simulink model "HARV_6DoF_turn_mdl"  (Simulink 9.3)
settings: Solver=ode45  StartTime=0.0  StopTime=100  FixedStep=0.01  MaxStep=0.01  MinStep=0.000001  RelTol=1e-3
model workspace (MAT data in the model file):
  op_trim1 : opcond.OperatingReport (value not decoded)
  op_trim3 : opcond.OperatingReport (value not decoded)
  op_trim5 : opcond.OperatingReport (value not decoded)
values from neighbouring files (symbols this model uses):
  b = 37.42*0.305    (= 11.4131)    [HARV_model.m]
  cbar = 11.52*0.305    (= 3.5136)    [HARV_model.m]
  GM = [c3 0 c4 0 c2 0 0 c1 0 ... (first row only)    [HARV_model.m]
  m = 1128.09*14.5939    (= 16463.232651)    [HARV_model.m]
  S = 400*(0.305^2)    (= 37.21)    [HARV_model.m]
undefined symbols (not defined in the file or in its folder): ad, ae, airlib, B747, DT, eqm, fms, gr, hlp
libraries: simulink x1
(part 1 of 2)
settings Model: Creator=kumabhi  LastModifiedBy=kumabhi
settings SolverCC: InitialStep=0.001  SolverJacobianMethodControl=SparsePerturbation
settings DataIOCC: ExternalInput=getinputstruct(op3)  InitialState=getstatestruct(op3)  LoadExternalInput=on  LoadInitialState=on  SignalLoggingSaveFormat=Dataset  SaveState=on  ReturnWorkspaceOutputs=on
settings OptimizationCC: LifeSpan=auto
settings DebuggingCC: UnderspecifiedInitializationDetection=Simplified  MergeDetectMultiDrivingBlocksExec=error  FcnCallInpInsideContextMsg=error  SFUnexpectedBacktrackingDiag=error  SFNoUnconditionalDefaultTransitionDiag=error  SFExecutionAtInitializationDiag=warning  ArithmeticOperatorsInVariantConditions=error
settings HardwareCC: ProdBitPerPointer=64  ProdBitPerSizeT=64  ProdBitPerPtrDiffT=64  ProdLargestAtomicFloat=Float  ProdIntDivRoundTo=Zero  ProdEndianess=LittleEndian  ProdWordSize=64  ProdHWDeviceType=Intel->x86-64 (Windows64)
settings ModelReferenceCC: PropagateSignalLabelsOutOfModel=on
settings SFSimCC: SimUseLocalCustomCode=on
settings RTWCC: RTWUseLocalCustomCode=on
settings CodeAppCC: StateflowObjectComments=off
settings GRTTargetCC: TargetLangStandard=C99 (ISO)  CombineOutputUpdateFcns=on  GRTInterface=off
settings ConfigComp: CovMetricSettings=dwe  CovHtmlReporting=off  CovSaveCumulativeToWorkspaceVar=off  CovSaveSingleToWorkspaceVar=off  CovExternalEMLEnable=on

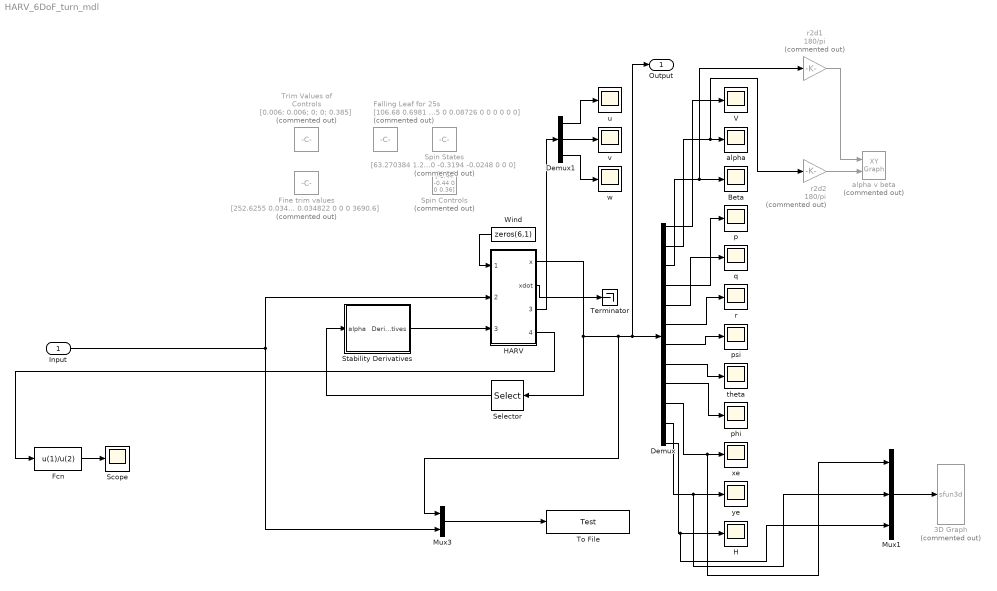
== system HARV_6DoF_turn_mdl ==
  Input : Inport
  3D Graph : S-Function  Commented=on  LoadFcn=if exist('sfun3d','file'), sfun3d([],[],[],'LoadBlock'); end  FunctionName=sfun3d  Parameters=ax,T,np,cp,gd,ls,mk,mx,hd,tb  SFunctionDeploymentMode=off  EnableBusSupport=off  mask(3D Graph){np=1, ax=[-300 3000 -3000 3000 -3000 3000], mx=1e7, T=0.1, cp=[3 2 1], gd=on, hd=off, tb=off, ls=-, mk=none}
      mask prompts: np "Number of moving points (lines)"; ax "Range: [xmin xmax  ymin ymax zmin zmax]"; mx "Max number of points in each line"; T "Sampling Time"; cp "Camera position (use [0 0 1] for 2D XY view)"; gd "Grid (on|off)"; hd "HeadMarkers (on|off)"; tb "Toolbar (on|off)"; ls "LineStyle"; mk "LineMarker"
      mask help:
      | This block plots the position of several points in the XYZ space. The input contains the coordinates of all the points (x1,y1,z1,x2,y2,z2,...).
      | The number of moving points (lines), the XYZ ranges, sampling time, camera position, and grid (among other things) can be set as mask parameters.
      settings: CopyFcn=if exist('sfun3d','file'), sfun3d([],[],[],'CopyBlock'); end  DeleteFcn=if exist('sfun3d','file'), sfun3d([],[],[],'DeleteBlock'); end  NameChangeFcn=if exist('sfun3d','file'), sfun3d([],[],[],'NameChange'); end
      mask Help:
      | This block plots the position of several points in the XYZ space. The input contains the coordinates of all the points (x1,y1,z1,x2,y2,z2,...).
      | The number of moving points (lines), the XYZ ranges, sampling time, camera position, and grid (among other things) can be set as mask parameters.
      mask TypeOptions ls: - | -- | : | -. | none
      mask TypeOptions mk: none | . | + | o | * | x | square | diamond | v | ^ | > | < | pentagram | hexagram
      mask Display: plot([.05 .95 .95 .05 .05],[.45 .45 .95 .95 .45], 0.5+cos(0:0.1:2*pi)*0.3,0.7+sin(0:0.1:2*pi)*0.2)
  Beta : Scope
  Demux : Demux  Outputs=12
  Demux1 : Demux  Outputs=3
  Falling Leaf for 25s : Constant  Commented=on  Value=[106.68 0.6981 0.349 0.1745 0 0.08726 0 0 0 0 0 0]
  Fcn : Fcn  Expr=u(1)/u(2)
  "Fine trim values " : Constant  Commented=on  Value=[252.6255 0.03482432 0 0 0 0 0 0.034822 0 0 0 3690.6]
  H : Scope
  HARV : Subsystem  AncestorBlock=airlib/DT-B747
  Mux1 : Mux  Inputs=3
  Mux3 : Mux  Inputs=2
  Scope : Scope
  Selector : Selector  InputPortWidth=12  IndexOptions=Index vector (dialog)  Indices=[2]  OutputSizes=1
  "Spin Controls " : Constant  Commented=on  Value=[-0.44 -0.44 0 0 0.36]
  "Spin States " : Constant  Commented=on  Value=[63.270384 1.2375 0.0382 -0.6163 0.1784 -1.4645 0 -0.3194 -0.0248 0 0 0]
  Stability Derivatives : Subsystem
  Terminator : Terminator
  To File : ToFile  Filename=Test  SaveFormat=Timeseries
  "Trim Values of Controls " : Constant  Commented=on  Value=[0.006; 0.006; 0; 0; 0.385]
  V : Scope
  Wind : Constant  Value=zeros(6,1)
  alpha : Scope
  alpha v beta : simulink/Sinks/XY Graph  Commented=on  xmin=-75  xmax=75  ymin=-30  ymax=80  st=-1
  p : Scope
  phi : Scope
  psi : Scope
  q : Scope
  r : Scope
  r2d1 : Gain  Commented=on  Gain=180/pi
  r2d2 : Gain  Commented=on  Gain=180/pi
  theta : Scope
  u : Scope
  v : Scope
  w : Scope
  xe : Scope
  ye : Scope
  Output : Outport
  wires:
  HARV/1(x) -> Mux3/1, Output/1, Demux/1, Selector/1
  Wind/1 -> HARV/1(Wind)
  Demux/1 -> V/1
  Demux/2 -> r2d2/1, alpha/1
  Demux/3 -> r2d1/1, Beta/1
  Demux/4 -> p/1
  Demux/5 -> q/1
  Demux/6 -> r/1
  Demux/7 -> psi/1
  Demux/8 -> theta/1
  Demux/11 -> Mux1/2, ye/1
  Demux/12 -> Mux1/3, H/1
  Demux/9 -> phi/1
  Demux/10 -> Mux1/1, xe/1
  HARV/3("[u v w]") -> Demux1/1
  Demux1/1 -> u/1
  Demux1/2 -> v/1
  Demux1/3 -> w/1
  HARV/2(xdot) -> Terminator/1
  Selector/1 -> Stability Derivatives/1(alpha)
  Stability Derivatives/1(Derivatives) -> HARV/3(Stability Derivatives)
  Mux1/1 -> 3D Graph/1
  r2d2/1 -> alpha v beta/2
  r2d1/1 -> alpha v beta/1
  Mux3/1 -> To File/1
  HARV/4(CAero) -> Fcn/1
  Input/1 -> HARV/2(Control), Mux3/2
  Fcn/1 -> Scope/1

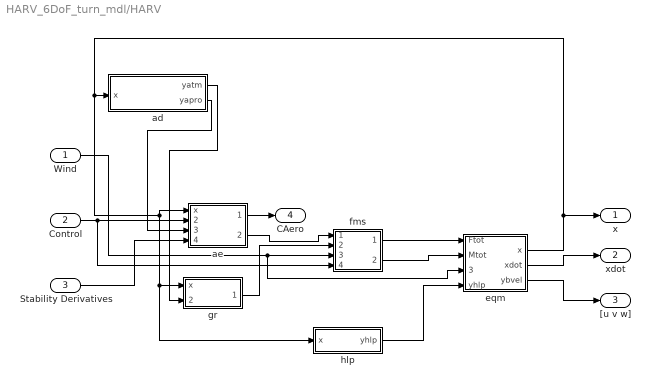
== system HARV_6DoF_turn_mdl/HARV ==
  Wind : Inport
  Control : Inport  Port=2
  Stability Derivatives : Inport  Port=3
  ad : Subsystem  AncestorBlock=airlib/DT-B747/ad
      mask Display: disp('ATMOSPHERE')
  ae : Subsystem  AncestorBlock=airlib/DT-B747/ae
      mask Display: disp('Faero')
  eqm : Subsystem  AncestorBlock=airlib/DT-B747/eqm
      mask Display: disp('ODE')
  fms : Subsystem  AncestorBlock=airlib/DT-B747/fms  mask(FMsort){}
      mask help: Forces and Moments sorting block
      mask Display: disp('FMsort')
  gr : Subsystem  AncestorBlock=airlib/DT-B747/gr  mask(Gravity){m=m}
      mask prompts: m "Mass of the aircraft [kg]:"
      mask help: Gravity forces.
      mask Display: disp('Gravity')
  hlp : Subsystem  AncestorBlock=airlib/DT-B747/hlp  mask(Hlpfcn){}
      mask help: Help sines and cosines
      mask Display: disp('hlpfcn')
  x : Outport
  xdot : Outport  Port=2
  "[u v w]" : Outport  Port=3
  CAero : Outport  Port=4
  wires:
  ad/2(yapro) -> ae/3(yaprop)
  Control/1 -> fms/4(Control), ae/2(Control)
  Stability Derivatives/1 -> ae/4(Stability Derivatives)
  ad/1(yatm) -> gr/2(yatm)
  ae/2(FMaero) -> fms/1(FMaero)
  Wind/1 -> eqm/3(uwind), fms/3(Fwind)
  gr/1(Fgrav) -> fms/2(Fgrav)
  ae/1(Caero) -> CAero/1
  fms/1(Ftot) -> eqm/1(Ftot)
  fms/2(Mtot) -> eqm/2(Mtot)
  hlp/1(yhlp) -> eqm/4(yhlp)
  eqm/1(x) -> hlp/1(x), gr/1(x), ae/1(x), ad/1(x), x/1
  eqm/2(xdot) -> xdot/1
  eqm/3(ybvel) -> "[u v w]"/1

== system HARV_6DoF_turn_mdl/Stability Derivatives ==
  alpha : Inport
  Lateral : Subsystem
  Longitudinal : Subsystem
  Mux : Mux  Inputs=2
  Derivatives : Outport
  wires:
  alpha/1 -> Longitudinal/1(alpha), Lateral/1(alpha)
  Lateral/1("CY, Cl, Cn") -> Mux/1
  Longitudinal/1("CL, CD, CM") -> Mux/2
  Mux/1 -> Derivatives/1

== system HARV_6DoF_turn_mdl/HARV/ad ==
  x : Inport
  ad1 : Subsystem  mask(Airdata1){}
      mask help: Basic airdata variables
      mask Display: disp('Airdata1')
  atm : Subsystem  mask(Atmosph){}
      mask help: Atmosphere variables
      mask Display: disp('Atmosph')
  yatm : Outport
  yapro : Outport  Port=2
  wires:
  ad1/1(yap) -> yapro/1
  atm/1(yatm) -> ad1/2(yatm), yatm/1
  x/1 -> ad1/1(x), atm/1(x)

== system HARV_6DoF_turn_mdl/HARV/ae ==
  x : Inport
  Control : Inport  Port=2
  yaprop : Inport  Port=3
  Stability Derivatives : Inport  Port=4
  ae : Subsystem  Commented=on  AncestorBlock=airlib/DT-B747/ae
  ae1 : Subsystem  AncestorBlock=airlib/DT-B747/ae
  ae2 : Subsystem  AncestorBlock=airlib/DT-B747/ae
  fmdims : Subsystem
      mask Display: disp('Forces & Moments')
  hlp : Subsystem  AncestorBlock=airlib/DT-B747/hlp  mask(Hlpfcn){}
      mask help: Help sines and cosines
      mask Display: disp('hlpfcn')
  Caero : Outport
  FMaero : Outport  Port=2
  wires:
  fmdims/1(Forces and moments) -> FMaero/1
  yaprop/1 -> ae2/2(ya), fmdims/1(yad1)
  Control/1 -> ae2/3(Controls)
  Stability Derivatives/1 -> ae2/1(Stability Derivatives)
  x/1 -> ae2/4(x), hlp/1(x)
  ae2/1(Output) -> ae1/1(Caero), Caero/1
  hlp/1(yhlp) -> ae1/2(helpfcn)
  ae1/1(CForce) -> fmdims/2(Force / moment derivatives)

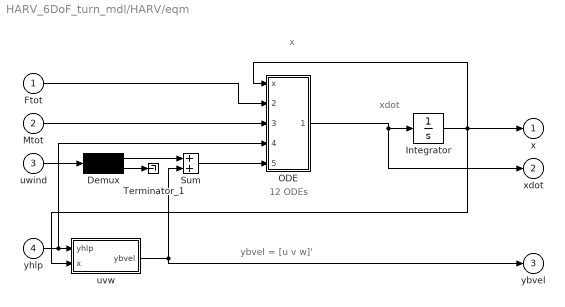
== system HARV_6DoF_turn_mdl/HARV/eqm ==
  note: 12 ODEs
  note: ybvel = [u v w]'
  note: x
  note: xdot
  Ftot : Inport
  Mtot : Inport  Port=2
  uwind : Inport  Port=3
  yhlp : Inport  Port=4
  Demux : Demux  Outputs=[3 3]
  Integrator : Integrator  InitialCondition=[54.7 0.5 0 -0.109 0.678 0.0538 0 0.9 0.9 0 0 0]
  ODE : Subsystem
  Sum : Sum  SaturateOnIntegerOverflow=on  InputSameDT=on  OutDataTypeStr=Inherit: Same as first input
  Terminator_1 : Terminator
  uvw : Subsystem  mask(uvw){}
      mask help:
      | Calculation of body-axes velocities
      | u, v, and w
      mask Display: disp('Body-axes\nvelocities')
  x : Outport
  xdot : Outport  Port=2
  ybvel : Outport  Port=3
  wires:
  ODE/1(xdot) -> Integrator/1, xdot/1
  Integrator/1 -> uvw/2(x), ODE/1(x), x/1
  Mtot/1 -> ODE/3(Mtot)
  Ftot/1 -> ODE/2(Ftot)
  Demux/1 -> Sum/1
  uwind/1 -> Demux/1
  uvw/1(ybvel) -> Sum/2, ybvel/1
  Sum/1 -> ODE/5(ybvel*)
  yhlp/1 -> ODE/4(yhlp), uvw/1(yhlp)
  Demux/2 -> Terminator_1/1

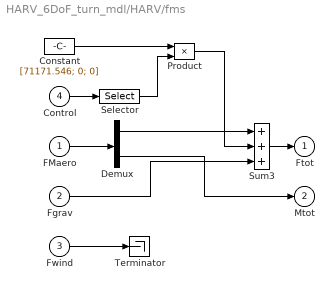
== system HARV_6DoF_turn_mdl/HARV/fms ==
  FMaero : Inport
  Fgrav : Inport  Port=2
  Fwind : Inport  Port=3
  Control : Inport  Port=4
  Constant : Constant  Value=[71171.546; 0; 0]
  Demux : Demux  Outputs=[3 3]
  Product : Product
  Selector : Selector  InputPortWidth=5  IndexOptions=Index vector (dialog)  Indices=[5]  OutputSizes=1
  Sum3 : Sum  Inputs=+++  SaturateOnIntegerOverflow=on  InputSameDT=on  OutDataTypeStr=Inherit: Same as first input
  Terminator : Terminator
  Ftot : Outport
  Mtot : Outport  Port=2
  wires:
  Demux/1 -> Sum3/1
  Demux/2 -> Mtot/1
  Sum3/1 -> Ftot/1
  Fgrav/1 -> Sum3/3
  FMaero/1 -> Demux/1
  Fwind/1 -> Terminator/1
  Control/1 -> Selector/1
  Selector/1 -> Product/2
  Constant/1 -> Product/1
  Product/1 -> Sum3/2

== system HARV_6DoF_turn_mdl/HARV/gr ==
  x : Inport
  yatm : Inport  Port=2
  Mux : Mux  Inputs=3
  Mux1 : Mux  Inputs=[12 5]
  Xgr : Fcn  Expr=-m*u[17]*sin(u[8])
  Ygr : Fcn  Expr=m*u[17]*cos(u[8])*sin(u[9])
  Zgr : Fcn  Expr=m*u[17]*cos(u[8])*cos(u[9])
  Fgrav : Outport
  wires:
  yatm/1 -> Mux1/2
  x/1 -> Mux1/1
  Zgr/1 -> Mux/3
  Mux1/1 -> Zgr/1, Xgr/1, Ygr/1
  Mux/1 -> Fgrav/1
  Ygr/1 -> Mux/2
  Xgr/1 -> Mux/1

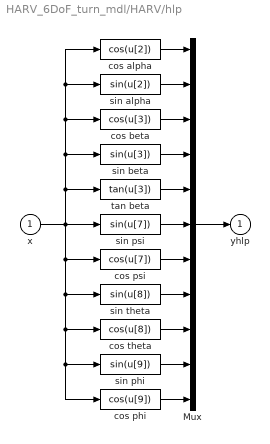
== system HARV_6DoF_turn_mdl/HARV/hlp ==
  x : Inport
  Mux : Mux  Inputs=11
  cos alpha : Fcn  Expr=cos(u[2])
  cos beta : Fcn  Expr=cos(u[3])
  cos phi : Fcn  Expr=cos(u[9])
  cos psi : Fcn  Expr=cos(u[7])
  cos theta : Fcn  Expr=cos(u[8])
  sin alpha : Fcn  Expr=sin(u[2])
  sin beta : Fcn  Expr=sin(u[3])
  sin phi : Fcn  Expr=sin(u[9])
  sin psi : Fcn  Expr=sin(u[7])
  sin theta : Fcn  Expr=sin(u[8])
  tan beta : Fcn  Expr=tan(u[3])
  yhlp : Outport
  wires:
  cos phi/1 -> Mux/11
  Mux/1 -> yhlp/1
  sin phi/1 -> Mux/10
  cos theta/1 -> Mux/9
  sin theta/1 -> Mux/8
  cos psi/1 -> Mux/7
  sin psi/1 -> Mux/6
  tan beta/1 -> Mux/5
  sin beta/1 -> Mux/4
  cos beta/1 -> Mux/3
  sin alpha/1 -> Mux/2
  cos alpha/1 -> Mux/1
  x/1 -> cos psi/1, cos phi/1, sin phi/1, cos theta/1, sin theta/1, tan beta/1, cos alpha/1, sin alpha/1, cos beta/1, sin beta/1, sin psi/1

== system HARV_6DoF_turn_mdl/Stability Derivatives/Lateral ==
  alpha : Inport
  CY : Subsystem
  Cl : Subsystem
  Cn : Subsystem
  Mux : Mux  Inputs=3
  "CY, Cl, Cn" : Outport
  wires:
  alpha/1 -> Cn/1(alpha), Cl/1(alpha), CY/1(alpha)
  Mux/1 -> "CY, Cl, Cn"/1
  CY/1(CY) -> Mux/1
  Cl/1(Cl) -> Mux/2
  Cn/1(Cn) -> Mux/3

== system HARV_6DoF_turn_mdl/Stability Derivatives/Longitudinal ==
  alpha : Inport
  CD : Subsystem
  CL : Subsystem
  CM : Subsystem
  Mux : Mux  Inputs=3
  "CL, CD, CM" : Outport
  wires:
  alpha/1 -> CD/1(Input), CL/1(alpha), CM/1(Input)
  CD/1(Output) -> Mux/1
  CL/1(CL_derivatives) -> Mux/2
  CM/1(Output) -> Mux/3
  Mux/1 -> "CL, CD, CM"/1

== system HARV_6DoF_turn_mdl/HARV/ad/ad1 ==
  x : Inport
  yatm : Inport  Port=2
  M : Fcn  Expr=u[2]/u[1]
  Mux : Mux  Inputs=[1 12]
  Mux1 : Mux  Inputs=[12 5]
  Mux2 : Mux  Inputs=3
  a : Fcn  Expr=sqrt(401.8743*u[3])
  qdyn : Fcn  Expr=0.5*u[13]*u[1]^2
  yap : Outport
  wires:
  yatm/1 -> Mux1/2, a/1
  x/1 -> Mux1/1, Mux/2
  Mux/1 -> M/1
  Mux1/1 -> qdyn/1
  M/1 -> Mux2/2
  a/1 -> Mux2/1, Mux/1
  qdyn/1 -> Mux2/3
  Mux2/1 -> yap/1

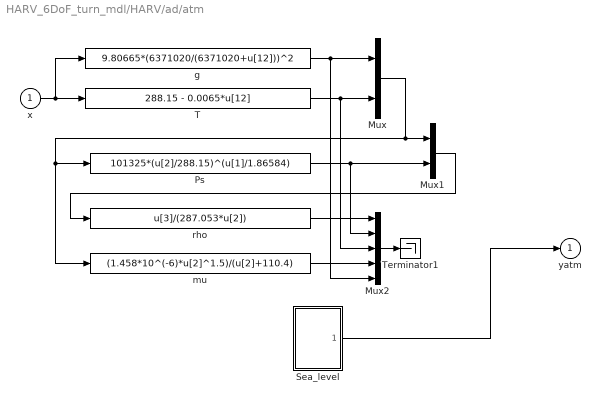
== system HARV_6DoF_turn_mdl/HARV/ad/atm ==
  x : Inport
  Mux : Mux  Inputs=2
  Mux1 : Mux  Inputs=[2 1]
  Mux2 : Mux  Inputs=5
  Ps : Fcn  Expr=101325*(u[2]/288.15)^(u[1]/1.86584)
  Sea_level : Subsystem
  T : Fcn  Expr=288.15 - 0.0065*u[12]
  Terminator1 : Terminator
  g : Fcn  Expr=9.80665*(6371020/(6371020+u[12]))^2
  mu : Fcn  Expr=(1.458*10^(-6)*u[2]^1.5)/(u[2]+110.4)
  rho : Fcn  Expr=u[3]/(287.053*u[2])
  yatm : Outport
  wires:
  mu/1 -> Mux2/4
  Mux1/1 -> rho/1
  rho/1 -> Mux2/1
  g/1 -> Mux2/5, Mux/1
  T/1 -> Mux2/3, Mux/2
  Ps/1 -> Mux2/2, Mux1/2
  Mux/1 -> Ps/1, mu/1, Mux1/1
  x/1 -> g/1, T/1
  Mux2/1 -> Terminator1/1
  Sea_level/1(Sea Level) -> yatm/1

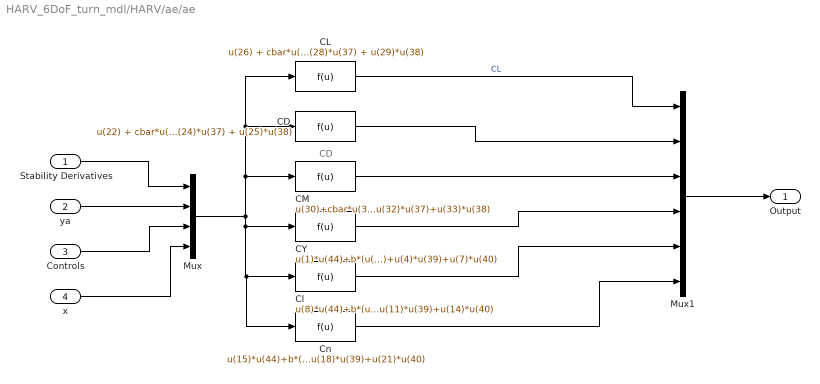
== system HARV_6DoF_turn_mdl/HARV/ae/ae ==
  note: CD
  Stability Derivatives : Inport
  ya : Inport  Port=2
  Controls : Inport  Port=3
  x : Inport  Port=4
  CD : Fcn  Expr=u(22) + cbar*u(23)*u(46)/(2*u(42))+ u(24)*u(37) + u(25)*u(38)
  CL : Fcn  Expr=u(26) + cbar*u(27)*u(46)/(2*u(42))+ u(28)*u(37) + u(29)*u(38)
  CM : Fcn  Expr=u(30)+cbar*u(31)*u(46)/(2*u(42))+u(32)*u(37)+u(33)*u(38)
  CY : Fcn  Expr=u(1)*u(44)+b*(u(2)*u(45)+u(3)*u(47))/(2*u(42))+u(4)*u(39)+u(7)*u(40)
  Cl : Fcn  Expr=u(8)*u(44)+b*(u(9)*u(45)+u(10)*u(47))/(2*u(42))+u(11)*u(39)+u(14)*u(40)
  Cn : Fcn  Expr=u(15)*u(44)+b*(u(16)*u(45)+u(17)*u(47))/(2*u(42))+u(18)*u(39)+u(21)*u(40)
  Mux : Mux
  Mux1 : Mux  Inputs=6
  Output : Outport
  wires:
  Stability Derivatives/1 -> Mux/1
  ya/1 -> Mux/2
  Mux/1 -> CM/1, CD/1, CL/1, Cn/1, Cl/1, CY/1
  Controls/1 -> Mux/3
  x/1 -> Mux/4
  CL/1 -> Mux1/1  "CL"
  CD/1 -> Mux1/2
  CM/1 -> Mux1/3
  CY/1 -> Mux1/4
  Cl/1 -> Mux1/5
  Cn/1 -> Mux1/6
  Mux1/1 -> Output/1

== system HARV_6DoF_turn_mdl/HARV/ae/ae1 ==
  Caero : Inport
  helpfcn : Inport  Port=2
  CX : Fcn  Expr=-u(2)*u(7)+u(1)*u(8)
  CZ : Fcn  Expr=-u(2)*u(8)-u(1)*u(7)
  Demux : Demux
  Mux : Mux  Inputs=2
  Mux1 : Mux  Inputs=6
  Selector : Selector  InputPortWidth=17  IndexOptions=Index vector (dialog)  Indices=[3:6]  OutputSizes=1
  CForce : Outport
  wires:
  Caero/1 -> Mux/1
  helpfcn/1 -> Mux/2
  Mux/1 -> Selector/1, CZ/1, CX/1
  CX/1 -> Mux1/1
  Mux1/1 -> CForce/1
  Selector/1 -> Demux/1
  CZ/1 -> Mux1/3
  Demux/2 -> Mux1/2
  Demux/3 -> Mux1/4
  Demux/1 -> Mux1/5
  Demux/4 -> Mux1/6

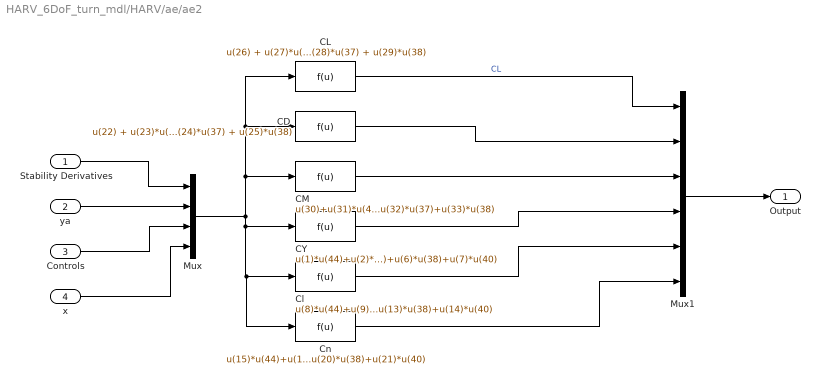
== system HARV_6DoF_turn_mdl/HARV/ae/ae2 ==
  Stability Derivatives : Inport
  ya : Inport  Port=2
  Controls : Inport  Port=3
  x : Inport  Port=4
  CD : Fcn  Expr=u(22) + u(23)*u(46)+ u(24)*u(37) + u(25)*u(38)
  CL : Fcn  Expr=u(26) + u(27)*u(46)+ u(28)*u(37) + u(29)*u(38)
  CM : Fcn  Expr=u(30)+u(31)*u(46)+u(32)*u(37)+u(33)*u(38)
  CY : Fcn  Expr=u(1)*u(44)+u(2)*u(45)+u(3)*u(47)+u(4)*u(39)+u(5)*u(37)+u(6)*u(38)+u(7)*u(40)
  Cl : Fcn  Expr=u(8)*u(44)+u(9)*u(45)+u(10)*u(47)+u(11)*u(39)+u(12)*u(37)+u(13)*u(38)+u(14)*u(40)
  Cn : Fcn  Expr=u(15)*u(44)+u(16)*u(45)+u(17)*u(47)+u(18)*u(39)+u(19)*u(37)+u(20)*u(38)+u(21)*u(40)
  Mux : Mux
  Mux1 : Mux  Inputs=6
  Output : Outport
  wires:
  Stability Derivatives/1 -> Mux/1
  ya/1 -> Mux/2
  Mux/1 -> CM/1, CD/1, CL/1, Cn/1, Cl/1, CY/1
  Controls/1 -> Mux/3
  x/1 -> Mux/4
  CL/1 -> Mux1/1  "CL"
  CD/1 -> Mux1/2
  CM/1 -> Mux1/3
  CY/1 -> Mux1/4
  Cl/1 -> Mux1/5
  Cn/1 -> Mux1/6
  Mux1/1 -> Output/1

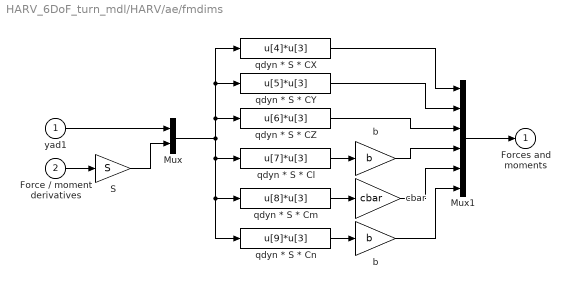
== system HARV_6DoF_turn_mdl/HARV/ae/fmdims ==
  yad1 : Inport
  Force / moment derivatives : Inport  Port=2
  Mux : Mux  Inputs=[3 6]
  Mux1 : Mux  Inputs=6
  S : Gain  Gain=S  SaturateOnIntegerOverflow=on  OutDataTypeStr=Inherit: Same as input  ParamDataTypeStr=Inherit: Same as input
  b : Gain  Gain=b  SaturateOnIntegerOverflow=on  OutDataTypeStr=Inherit: Same as input  ParamDataTypeStr=Inherit: Same as input
  "b " : Gain  Gain=b  SaturateOnIntegerOverflow=on  OutDataTypeStr=Inherit: Same as input  ParamDataTypeStr=Inherit: Same as input
  cbar : Gain  Gain=cbar  SaturateOnIntegerOverflow=on  OutDataTypeStr=Inherit: Same as input  ParamDataTypeStr=Inherit: Same as input
  qdyn * S * CX : Fcn  Expr=u[4]*u[3]
  qdyn * S * CY : Fcn  Expr=u[5]*u[3]
  qdyn * S * CZ : Fcn  Expr=u[6]*u[3]
  qdyn * S * Cl : Fcn  Expr=u[7]*u[3]
  qdyn * S * Cm : Fcn  Expr=u[8]*u[3]
  qdyn * S * Cn : Fcn  Expr=u[9]*u[3]
  Forces and moments : Outport
  wires:
  b/1 -> Mux1/4
  qdyn * S * CZ/1 -> Mux1/3
  S/1 -> Mux/2
  qdyn * S * CY/1 -> Mux1/2
  qdyn * S * CX/1 -> Mux1/1
  yad1/1 -> Mux/1
  qdyn * S * Cn/1 -> "b "/1
  qdyn * S * Cm/1 -> cbar/1
  qdyn * S * Cl/1 -> b/1
  Mux/1 -> qdyn * S * Cn/1, qdyn * S * Cm/1, qdyn * S * Cl/1, qdyn * S * CY/1, qdyn * S * CX/1, qdyn * S * CZ/1
  Force / moment derivatives/1 -> S/1
  cbar/1 -> Mux1/5
  "b "/1 -> Mux1/6
  Mux1/1 -> Forces and moments/1

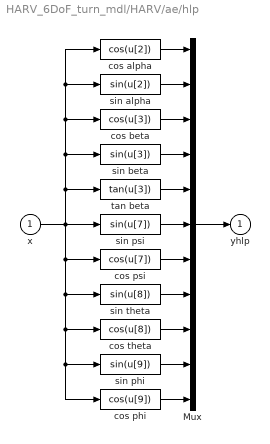
== system HARV_6DoF_turn_mdl/HARV/ae/hlp ==
  x : Inport
  Mux : Mux  Inputs=11
  cos alpha : Fcn  Expr=cos(u[2])
  cos beta : Fcn  Expr=cos(u[3])
  cos phi : Fcn  Expr=cos(u[9])
  cos psi : Fcn  Expr=cos(u[7])
  cos theta : Fcn  Expr=cos(u[8])
  sin alpha : Fcn  Expr=sin(u[2])
  sin beta : Fcn  Expr=sin(u[3])
  sin phi : Fcn  Expr=sin(u[9])
  sin psi : Fcn  Expr=sin(u[7])
  sin theta : Fcn  Expr=sin(u[8])
  tan beta : Fcn  Expr=tan(u[3])
  yhlp : Outport
  wires:
  cos phi/1 -> Mux/11
  Mux/1 -> yhlp/1
  sin phi/1 -> Mux/10
  cos theta/1 -> Mux/9
  sin theta/1 -> Mux/8
  cos psi/1 -> Mux/7
  sin psi/1 -> Mux/6
  tan beta/1 -> Mux/5
  sin beta/1 -> Mux/4
  cos beta/1 -> Mux/3
  sin alpha/1 -> Mux/2
  cos alpha/1 -> Mux/1
  x/1 -> cos psi/1, cos phi/1, sin phi/1, cos theta/1, sin theta/1, tan beta/1, cos alpha/1, sin alpha/1, cos beta/1, sin beta/1, sin psi/1

== system HARV_6DoF_turn_mdl/HARV/eqm/ODE ==
  x : Inport
  Ftot : Inport  Port=2
  Mtot : Inport  Port=3
  yhlp : Inport  Port=4
  ybvel* : Inport  Port=5
  Eulerdot : Subsystem  mask(Eulerdot){}
      mask help:
      | Calculation of d(psi)/dt, d(theta)/dt,
      | and d(phi/dt)
      mask Display: disp('psi dot\ntheta dot\nphi dot')
  Mux : Mux  Inputs=[12 3 3 11]
  Mux1 : Mux  Inputs=[3 3 3 3]
  Vabdot : Subsystem  mask(Vabdot){}
      mask help: Calculation of dV/dt, dalpha/dt, dbeta/dt.
      mask Display: disp('V dot\nalpha dot\nbeta dot')
  pqrdot : Subsystem  mask(pqrdot){}
      mask help: Calculation of dp/dt, dq/dt, and dr/dt
      mask Display: disp('p dot\nq dot\nr dot')
  xyHdot : Subsystem  mask(xyHdot){}
      mask help: Calculation of d(xe)/dt, d(ye)/dt, and dH/dt
      mask Display: disp('xe dot\nye dot\nH dot')
  xdot : Outport
  wires:
  Mux1/1 -> xdot/1
  Vabdot/1(yVab) -> Mux1/1
  pqrdot/1(ypqr) -> Mux1/2
  Eulerdot/1(yeul) -> Mux1/3
  xyHdot/1(yxyH) -> Mux1/4
  yhlp/1 -> Mux/4
  ybvel*/1 -> xyHdot/1(ybvel*)
  Mux/1 -> xyHdot/2(uxYH), Eulerdot/1(ueul), Vabdot/1(uVab), pqrdot/1(upqr)
  Ftot/1 -> Mux/2
  Mtot/1 -> Mux/3
  x/1 -> Mux/1

== system HARV_6DoF_turn_mdl/HARV/eqm/uvw ==
  yhlp : Inport
  x : Inport  Port=2
  Mux : Mux  Inputs=3
  Mux1 : Mux  Inputs=[12 11]
  u : Fcn  Expr=u[1]*u[13]*u[15]
  v : Fcn  Expr=u[1]*u[16]
  w : Fcn  Expr=u[1]*u[14]*u[15]
  ybvel : Outport
  wires:
  Mux/1 -> ybvel/1
  w/1 -> Mux/3
  v/1 -> Mux/2
  u/1 -> Mux/1
  x/1 -> Mux1/1
  yhlp/1 -> Mux1/2
  Mux1/1 -> v/1, w/1, u/1

== system HARV_6DoF_turn_mdl/Stability Derivatives/Lateral/CY ==
  alpha : Inport
  CY_b : Lookup_n-D  NumberOfTableDimensions=1  BreakpointsForDimension1=[-0.2444,-0.1746,-0.1048,-0.0349,0.0349,0.1048,0.1746,0.2444,0.3143,0.3841,0.4540,0.5238,0.5937,0.6635,0.7333,0.8032,0.8730,0.9429,1.0127,1.0825,1.1524,1.2222,1.2921,1.3619,1.4317,1.5016,1.5714]  Table=[-0.9848,-0.9848,-1.0161,-1.0473,-1.0549,-1.0547,-1.0754,-1.0145,-0.8881,-0.8074,-0.7265,-0.7373,-0.7168,-0.7766,-0.8036,-0.7625,-0.6844,0.7484,-0.7853,-0.7877,-0.7642,-0.7393,-0.7622,-0.7922,-0.7893,-0.7544,-0.7294]  InternalRulePriority=Speed  RndMeth=Simplest  InputSameDT=on
  CY_da : Lookup_n-D  NumberOfTableDimensions=1  BreakpointsForDimension1=[-0.2444,-0.1746,-0.1048,-0.0349,0.0349,0.1048,0.1746,0.2444,0.3143,0.3841,0.4540,0.5238,0.5937,0.6635,0.7333,0.8032,0.8730,0.9429,1.0127,1.0825,1.1524,1.2222,1.2921,1.3619,1.4317,1.5016,1.5714]  Table=|  InternalRulePriority=Speed  RndMeth=Simplest  InputSameDT=on
      | [
      |    -0.0331,
      |    -0.0331,
      |    -0.0331,
      |    -0.0313,
      |    -0.0264,
      |    -0.0233,
      |    -0.0238,
      |    -0.0212,
      |    -0.0112,
      |     0.0026,
      |     0.0151,
      |     0.0271,
      |     0.0366,
      |     0.0406,
      |     0.0372,
      |     0.0114,
      |    -0.0058,
      |    -0.0085,
      |    -0.0100,
      |    -0.0112,
      |    -0.0125,
      |    -0.0138,
      |    -0.0159,
      |    -0.0175,
      |    -0.0188,
      |    -0.0199,
      |    -0.0210]
  CY_da1 : Lookup_n-D  Commented=on  NumberOfTableDimensions=1  BreakpointsForDimension1=[-0.2444,-0.1746,-0.1048,-0.0349,0.0349,0.1048,0.1746,0.2444,0.3143,0.3841,0.4540,0.5238,0.5937,0.6635,0.7333,0.8032,0.8730,0.9429,1.0127,1.0825,1.1524,1.2222,1.2921,1.3619,1.4317,1.5016,1.5714]  Table=[0,0,0,0,0,0,0,0,0,0,0,0,0,0,0,0,0,0,0,0,0,0,0,0,0,0,0]  InternalRulePriority=Speed  RndMeth=Simplest  InputSameDT=on
  CY_del : Lookup_n-D  NumberOfTableDimensions=1  BreakpointsForDimension1=[-0.2444,-0.1746,-0.1048,-0.0349,0.0349,0.1048,0.1746,0.2444,0.3143,0.3841,0.4540,0.5238,0.5937,0.6635,0.7333,0.8032,0.8730,0.9429,1.0127,1.0825,1.1524,1.2222,1.2921,1.3619,1.4317,1.5016,1.5714]  Table=|  InternalRulePriority=Speed  RndMeth=Simplest  InputSameDT=on
      | [   -0.0698,
      |    -0.0698,
      |    -0.0698,
      |    -0.0679,
      |    -0.0622,
      |    -0.0555,
      |    -0.0494,
      |    -0.0403,
      |    -0.0286,
      |    -0.0165,
      |    -0.0029,
      |     0.0118,
      |     0.0245,
      |     0.0339,
      |     0.0416,
      |     0.0491,
      |     0.0576,
      |     0.0648,
      |     0.0703,
      |     0.0747,
      |     0.0743,
      |     0.0616,
      |     0.0289,
      |    -0.0026,
      |    -0.0326,
      |    -0.0573,
      |    -0.0693]
  CY_der : Lookup_n-D  NumberOfTableDimensions=1  BreakpointsForDimension1=[-0.2444,-0.1746,-0.1048,-0.0349,0.0349,0.1048,0.1746,0.2444,0.3143,0.3841,0.4540,0.5238,0.5937,0.6635,0.7333,0.8032,0.8730,0.9429,1.0127,1.0825,1.1524,1.2222,1.2921,1.3619,1.4317,1.5016,1.5714]  Table=|  InternalRulePriority=Speed  RndMeth=Simplest  InputSameDT=on
      | [    0.0698,
      |     0.0698,
      |     0.0698,
      |     0.0679,
      |     0.0622,
      |     0.0555,
      |     0.0494,
      |     0.0403,
      |     0.0286,
      |     0.0165,
      |     0.0029,
      |    -0.0118,
      |    -0.0245,
      |    -0.0339,
      |    -0.0416,
      |    -0.0491,
      |    -0.0576,
      |    -0.0648,
      |    -0.0703,
      |    -0.0747,
      |    -0.0743,
      |    -0.0616,
      |    -0.0289,
      |     0.0026,
      |     0.0326,
      |     0.0573,
      |     0.0693]
  CY_dr : Lookup_n-D  NumberOfTableDimensions=1  BreakpointsForDimension1=[-0.2444,-0.1746,-0.1048,-0.0349,0.0349,0.1048,0.1746,0.2444,0.3143,0.3841,0.4540,0.5238,0.5937,0.6635,0.7333,0.8032,0.8730,0.9429,1.0127,1.0825,1.1524,1.2222,1.2921,1.3619,1.4317,1.5016,1.5714]  Table=|  InternalRulePriority=Speed  RndMeth=Simplest  InputSameDT=on
      | [
      |     0.1984,
      |     0.1984,
      |     0.1984,
      |     0.2022,
      |     0.2101,
      |     0.2138,
      |     0.2101,
      |     0.1984,
      |     0.1765,
      |     0.1477,
      |     0.1211,
      |     0.1029,
      |     0.0913,
      |     0.0843,
      |     0.0865,
      |     0.0915,
      |     0.0849,
      |     0.0721,
      |     0.0598,
      |     0.0557,
      |     0.0600,
      |     0.0661,
      |     0.0631,
      |     0.0581,
      |     0.0600,
      |     0.0660,
      |     0.0621]
  CY_p : Lookup_n-D  NumberOfTableDimensions=1  BreakpointsForDimension1=[-0.2444,-0.1746,-0.1048,-0.0349,0.0349,0.1048,0.1746,0.2444,0.3143,0.3841,0.4540,0.5238,0.5937,0.6635,0.7333,0.8032,0.8730,0.9429,1.0127,1.0825,1.1524,1.2222,1.2921,1.3619,1.4317,1.5016,1.5714]  Table=|  InternalRulePriority=Speed  RndMeth=Simplest  InputSameDT=on
      | [   -0.0610,
      |    -0.0610,
      |    -0.0610,
      |    -0.0495,
      |    -0.0120,
      |     0.0237,
      |     0.0332,
      |     0.0305,
      |     0.0260,
      |     0.0127,
      |    -0.0100,
      |    -0.0315,
      |    -0.0540,
      |    -0.0777,
      |    -0.1493,
      |    -0.2519,
      |    -0.2999,
      |    -0.1719,
      |    -0.0950,
      |    -0.0450,
      |    -0.0170,
      |    -0.0250,
      |    -0.0530,
      |    -0.0570,
      |    -0.0530,
      |    -0.0560,
      |    -0.0800]
  CY_r : Lookup_n-D  NumberOfTableDimensions=1  BreakpointsForDimension1=[-0.2444,-0.1746,-0.1048,-0.0349,0.0349,0.1048,0.1746,0.2444,0.3143,0.3841,0.4540,0.5238,0.5937,0.6635,0.7333,0.8032,0.8730,0.9429,1.0127,1.0825,1.1524,1.2222,1.2921,1.3619,1.4317,1.5016,1.5714]  Table=[0.1544,0.1544,0.1544,0.1659,0.1927,0.2259,0.2554,0.2189,0.0702,-0.0925,-0.1984,-0.2674,-0.3074,-0.3249,-0.2229,0.0020,0.2899,0.2899,0.2359,0.1599,0.0920,0.0600,0.0480,0.0360,0.0280,0.0240,0.0200]  InternalRulePriority=Speed  RndMeth=Simplest  InputSameDT=on
  Mux : Mux  Inputs=7
  CY : Outport
  wires:
  alpha/1 -> CY_p/1, CY_b/1, CY_r/1, CY_del/1, CY_der/1, CY_dr/1, CY_da/1
  CY_b/1 -> Mux/1
  CY_p/1 -> Mux/2
  CY_r/1 -> Mux/3
  CY_da/1 -> Mux/4
  CY_dr/1 -> Mux/7
  Mux/1 -> CY/1
  CY_del/1 -> Mux/5
  CY_der/1 -> Mux/6

== system HARV_6DoF_turn_mdl/Stability Derivatives/Lateral/Cl ==
  alpha : Inport
  Cl_b : Lookup_n-D  NumberOfTableDimensions=1  BreakpointsForDimension1=[-0.2444,-0.1746,-0.1048,-0.0349,0.0349,0.1048,0.1746,0.2444,0.3143,0.3841,0.4540,0.5238,0.5937,0.6635,0.7333,0.8032,0.8730,0.9429,1.0127,1.0825,1.1524,1.2222,1.2921,1.3619,1.4317,1.5016,1.5714]  Table=|  InternalRulePriority=Speed  RndMeth=Simplest  InputSameDT=on
      | [   -0.0021,
      |    -0.0021,
      |    -0.0253,
      |    -0.0485,
      |    -0.0728,
      |    -0.0974,
      |    -0.1210,
      |    -0.1587,
      |    -0.1932,
      |    -0.1992,
      |    -0.1813,
      |    -0.1350,
      |    -0.0702,
      |    -0.0656,
      |    -0.0938,
      |    -0.1277,
      |    -0.1408,
      |    -0.1419,
      |    -0.1400,
      |    -0.1441,
      |    -0.1552,
      |    -0.1666,
      |    -0.1619,
      |    -0.1579,
      |    -0.1550,
      |    -0.1531,
      |    -0.1524]
  Cl_da : Lookup_n-D  NumberOfTableDimensions=1  BreakpointsForDimension1=[-0.2444,-0.1746,-0.1048,-0.0349,0.0349,0.1048,0.1746,0.2444,0.3143,0.3841,0.4540,0.5238,0.5937,0.6635,0.7333,0.8032,0.8730,0.9429,1.0127,1.0825,1.1524,1.2222,1.2921,1.3619,1.4317,1.5016,1.5714]  Table=|  InternalRulePriority=Speed  RndMeth=Simplest  InputSameDT=on
      | [    0.0667,
      |     0.0667,
      |     0.0667,
      |     0.0668,
      |     0.0670,
      |     0.0673,
      |     0.0653,
      |     0.0596,
      |     0.0481,
      |     0.0362,
      |     0.0300,
      |     0.0262,
      |     0.0221,
      |     0.0183,
      |     0.0161,
      |     0.0147,
      |     0.0134,
      |     0.0121,
      |     0.0113,
      |     0.0107,
      |     0.0100,
      |     0.0089,
      |     0.0055,
      |     0.0029,
      |     0.0010,
      |    -0.0000,
      |    -0.0000]
  Cl_del : Lookup_n-D  NumberOfTableDimensions=1  BreakpointsForDimension1=[-0.2444,-0.1746,-0.1048,-0.0349,0.0349,0.1048,0.1746,0.2444,0.3143,0.3841,0.4540,0.5238,0.5937,0.6635,0.7333,0.8032,0.8730,0.9429,1.0127,1.0825,1.1524,1.2222,1.2921,1.3619,1.4317,1.5016,1.5714]  Table=|  InternalRulePriority=Speed  RndMeth=Simplest  InputSameDT=on
      | [
      |     0.0324,
      |     0.0324,
      |     0.0324,
      |     0.0332,
      |     0.0351,
      |     0.0371,
      |     0.0389,
      |     0.0395,
      |     0.0393,
      |     0.0395,
      |     0.0400,
      |     0.0400,
      |     0.0391,
      |     0.0373,
      |     0.0341,
      |     0.0297,
      |     0.0248,
      |     0.0197,
      |     0.0153,
      |     0.0116,
      |     0.0082,
      |     0.0047,
      |     0.0014,
      |    -0.0003,
      |    -0.0017,
      |    -0.0032,
      |    -0.0046]
  Cl_der : Lookup_n-D  NumberOfTableDimensions=1  BreakpointsForDimension1=[-0.2444,-0.1746,-0.1048,-0.0349,0.0349,0.1048,0.1746,0.2444,0.3143,0.3841,0.4540,0.5238,0.5937,0.6635,0.7333,0.8032,0.8730,0.9429,1.0127,1.0825,1.1524,1.2222,1.2921,1.3619,1.4317,1.5016,1.5714]  Table=|  InternalRulePriority=Speed  RndMeth=Simplest  InputSameDT=on
      | [   -0.0324,
      |    -0.0324,
      |    -0.0324,
      |    -0.0332,
      |    -0.0351,
      |    -0.0371,
      |    -0.0389,
      |    -0.0395,
      |    -0.0393,
      |    -0.0395,
      |    -0.0400,
      |    -0.0400,
      |    -0.0391,
      |    -0.0373,
      |    -0.0341,
      |    -0.0297,
      |    -0.0248,
      |    -0.0197,
      |    -0.0153,
      |    -0.0116,
      |    -0.0082,
      |    -0.0047,
      |    -0.0014,
      |     0.0003,
      |     0.0017,
      |     0.0032,
      |     0.0046]
  Cl_dr : Lookup_n-D  NumberOfTableDimensions=1  BreakpointsForDimension1=[-0.2444,-0.1746,-0.1048,-0.0349,0.0349,0.1048,0.1746,0.2444,0.3143,0.3841,0.4540,0.5238,0.5937,0.6635,0.7333,0.8032,0.8730,0.9429,1.0127,1.0825,1.1524,1.2222,1.2921,1.3619,1.4317,1.5016,1.5714]  Table=[0.0164,0.0164,0.0164,0.0154,0.0137,0.0125,0.0121,0.0119,0.0103,0.0071,0.0040,0.0020,0.0011,0.0003,-0.0020,-0.0050,-0.0062,-0.0045,-0.0015,0.0021,0.0054,0.0072,0.0055,0.0044,0.0039,0.0037,0.0036]  InternalRulePriority=Speed  RndMeth=Simplest  InputSameDT=on
  Cl_p : Lookup_n-D  NumberOfTableDimensions=1  BreakpointsForDimension1=[-0.2444,-0.1746,-0.1048,-0.0349,0.0349,0.1048,0.1746,0.2444,0.3143,0.3841,0.4540,0.5238,0.5937,0.6635,0.7333,0.8032,0.8730,0.9429,1.0127,1.0825,1.1524,1.2222,1.2921,1.3619,1.4317,1.5016,1.5714]  Table=|  InternalRulePriority=Speed  RndMeth=Simplest  InputSameDT=on
      | [   -0.4038,
      |    -0.4038,
      |    -0.4038,
      |    -0.4038,
      |    -0.4038,
      |    -0.4038,
      |    -0.3579,
      |    -0.3009,
      |    -0.2649,
      |    -0.2209,
      |    -0.3084,
      |    -0.4548,
      |    -0.4973,
      |    -0.4998,
      |    -0.2799,
      |     0.0020,
      |    -0.1899,
      |    -0.2139,
      |    -0.2319,
      |    -0.2499,
      |    -0.2679,
      |    -0.2799,
      |    -0.2879,
      |    -0.2959,
      |    -0.3039,
      |    -0.3099,
      |    -0.3099]
  Cl_r : Lookup_n-D  NumberOfTableDimensions=1  BreakpointsForDimension1=[-0.2444,-0.1746,-0.1048,-0.0349,0.0349,0.1048,0.1746,0.2444,0.3143,0.3841,0.4540,0.5238,0.5937,0.6635,0.7333,0.8032,0.8730,0.9429,1.0127,1.0825,1.1524,1.2222,1.2921,1.3619,1.4317,1.5016,1.5714]  Table=|  InternalRulePriority=Speed  RndMeth=Simplest  InputSameDT=on
      | [    0.0123,
      |     0.0123,
      |     0.0123,
      |     0.0335,
      |     0.0875,
      |     0.1472,
      |     0.1942,
      |     0.2202,
      |     0.2285,
      |     0.2357,
      |     0.2539,
      |     0.2972,
      |     0.3254,
      |     0.2902,
      |     0.2333,
      |     0.1879,
      |     0.1467,
      |     0.1251,
      |     0.1066,
      |     0.0906,
      |     0.0766,
      |     0.0638,
      |     0.0646,
      |     0.0648,
      |     0.0532,
      |     0.0306,
      |     0.0098]
  Mux : Mux  Inputs=7
  Cl : Outport
  wires:
  alpha/1 -> Cl_dr/1, Cl_der/1, Cl_del/1, Cl_p/1, Cl_b/1, Cl_r/1, Cl_da/1
  Cl_b/1 -> Mux/1
  Cl_p/1 -> Mux/2
  Cl_r/1 -> Mux/3
  Cl_da/1 -> Mux/4
  Cl_del/1 -> Mux/5
  Cl_der/1 -> Mux/6
  Cl_dr/1 -> Mux/7
  Mux/1 -> Cl/1

== system HARV_6DoF_turn_mdl/Stability Derivatives/Lateral/Cn ==
  alpha : Inport
  CY_da1 : Lookup_n-D  Commented=on  NumberOfTableDimensions=1  BreakpointsForDimension1=[-0.2444,-0.1746,-0.1048,-0.0349,0.0349,0.1048,0.1746,0.2444,0.3143,0.3841,0.4540,0.5238,0.5937,0.6635,0.7333,0.8032,0.8730,0.9429,1.0127,1.0825,1.1524,1.2222,1.2921,1.3619,1.4317,1.5016,1.5714]  Table=[0,0,0,0,0,0,0,0,0,0,0,0,0,0,0,0,0,0,0,0,0,0,0,0,0,0,0]  InternalRulePriority=Speed  RndMeth=Simplest  InputSameDT=on
  Cn_b : Lookup_n-D  NumberOfTableDimensions=1  BreakpointsForDimension1=[-0.2444,-0.1746,-0.1048,-0.0349,0.0349,0.1048,0.1746,0.2444,0.3143,0.3841,0.4540,0.5238,0.5937,0.6635,0.7333,0.8032,0.8730,0.9429,1.0127,1.0825,1.1524,1.2222,1.2921,1.3619,1.4317,1.5016,1.5714]  Table=|  InternalRulePriority=Speed  RndMeth=Simplest  InputSameDT=on
      | [    0.0814,
      |     0.0814,
      |     0.0874,
      |     0.0933,
      |     0.0946,
      |     0.0957,
      |     0.1031,
      |     0.0836,
      |     0.0568,
      |     0.0391,
      |     0.0101,
      |    -0.0625,
      |    -0.0636,
      |    -0.0913,
      |    -0.1081,
      |    -0.1012,
      |    -0.0778,
      |    -0.0875,
      |    -0.0935,
      |    -0.0911,
      |    -0.0827,
      |    -0.0770,
      |    -0.0846,
      |    -0.0921,
      |    -0.0971,
      |    -0.0990,
      |    -0.0995]
  Cn_da : Lookup_n-D  NumberOfTableDimensions=1  BreakpointsForDimension1=[-0.2444,-0.1746,-0.1048,-0.0349,0.0349,0.1048,0.1746,0.2444,0.3143,0.3841,0.4540,0.5238,0.5937,0.6635,0.7333,0.8032,0.8730,0.9429,1.0127,1.0825,1.1524,1.2222,1.2921,1.3619,1.4317,1.5016,1.5714]  Table=|  InternalRulePriority=Speed  RndMeth=Simplest  InputSameDT=on
      | [   -0.0005,
      |    -0.0005,
      |    -0.0005,
      |    -0.0012,
      |    -0.0020,
      |    -0.0023,
      |    -0.0027,
      |    -0.0035,
      |    -0.0044,
      |    -0.0059,
      |    -0.0076,
      |    -0.0089,
      |    -0.0099,
      |    -0.0103,
      |    -0.0113,
      |    -0.0118,
      |    -0.0138,
      |    -0.0154,
      |    -0.0165,
      |    -0.0173,
      |    -0.0063,
      |     0.0000,
      |     0.0048,
      |     0.0091,
      |     0.0127,
      |     0.0140,
      |     0.0100]
  Cn_del : Lookup_n-D  NumberOfTableDimensions=1  BreakpointsForDimension1=[-0.2444,-0.1746,-0.1048,-0.0349,0.0349,0.1048,0.1746,0.2444,0.3143,0.3841,0.4540,0.5238,0.5937,0.6635,0.7333,0.8032,0.8730,0.9429,1.0127,1.0825,1.1524,1.2222,1.2921,1.3619,1.4317,1.5016,1.5714]  Table=|  InternalRulePriority=Speed  RndMeth=Simplest  InputSameDT=on
      | [    0.0255,
      |     0.0255,
      |     0.0255,
      |     0.0250,
      |     0.0239,
      |     0.0226,
      |     0.0205,
      |     0.0162,
      |     0.0096,
      |     0.0037,
      |    -0.0005,
      |    -0.0052,
      |    -0.0117,
      |    -0.0191,
      |    -0.0246,
      |    -0.0273,
      |    -0.0260,
      |    -0.0300,
      |    -0.0367,
      |    -0.0457,
      |    -0.0565,
      |    -0.0690,
      |    -0.0881,
      |    -0.1130,
      |    -0.1324,
      |    -0.1441,
      |    -0.1550]
  Cn_der : Lookup_n-D  NumberOfTableDimensions=1  BreakpointsForDimension1=[-0.2444,-0.1746,-0.1048,-0.0349,0.0349,0.1048,0.1746,0.2444,0.3143,0.3841,0.4540,0.5238,0.5937,0.6635,0.7333,0.8032,0.8730,0.9429,1.0127,1.0825,1.1524,1.2222,1.2921,1.3619,1.4317,1.5016,1.5714]  Table=[-0.0255,-0.0255,-0.0255,-0.0250,-0.0239,-0.0226,-0.0205,-0.0162,-0.0096,-0.0037,0.0005,0.0052,0.0117,0.0191,0.0265,0.0338,0.0434,0.0505,0.0591,0.0675,0.0760,0.0869,0.1057,0.1255,0.1386,0.1454,0.1550]  InternalRulePriority=Speed  RndMeth=Simplest  InputSameDT=on
  Cn_dr : Lookup_n-D  NumberOfTableDimensions=1  BreakpointsForDimension1=[-0.2444,-0.1746,-0.1048,-0.0349,0.0349,0.1048,0.1746,0.2444,0.3143,0.3841,0.4540,0.5238,0.5937,0.6635,0.7333,0.8032,0.8730,0.9429,1.0127,1.0825,1.1524,1.2222,1.2921,1.3619,1.4317,1.5016,1.5714]  Table=[-0.0661,-0.0661,-0.0661,-0.0668,-0.0677,-0.0677,-0.0662,-0.0620,-0.0549,-0.0460,-0.0390,-0.0354,-0.0338,-0.0333,-0.0295,-0.0239,-0.0213,-0.0222,-0.0221,-0.0201,-0.0172,-0.0158,-0.0155,-0.0185,-0.0220,-0.0242,-0.0239]  InternalRulePriority=Speed  RndMeth=Simplest  InputSameDT=on
  Cn_p : Lookup_n-D  NumberOfTableDimensions=1  BreakpointsForDimension1=[-0.2444,-0.1746,-0.1048,-0.0349,0.0349,0.1048,0.1746,0.2444,0.3143,0.3841,0.4540,0.5238,0.5937,0.6635,0.7333,0.8032,0.8730,0.9429,1.0127,1.0825,1.1524,1.2222,1.2921,1.3619,1.4317,1.5016,1.5714]  Table=[-0.0724,-0.0724,-0.0724,-0.0708,-0.0675,-0.0642,-0.0538,-0.0365,-0.0142,0.0057,0.0212,0.0262,0.0227,0.0142,0.0134,0.0240,0.0400,0.0560,-0.0600,-0.0920,-0.0186,-0.0130,-0.0826,-0.0400,-0.0000,-0.0000,-0.0000]  InternalRulePriority=Speed  RndMeth=Simplest  InputSameDT=on
  Cn_r : Lookup_n-D  NumberOfTableDimensions=1  BreakpointsForDimension1=[-0.2444,-0.1746,-0.1048,-0.0349,0.0349,0.1048,0.1746,0.2444,0.3143,0.3841,0.4540,0.5238,0.5937,0.6635,0.7333,0.8032,0.8730,0.9429,1.0127,1.0825,1.1524,1.2222,1.2921,1.3619,1.4317,1.5016,1.5714]  Table=[-0.1787,-0.1787,-0.1787,-0.1782,-0.1779,-0.1792,-0.1819,-0.1877,-0.1984,-0.2279,-0.2651,-0.2949,-0.3169,-0.3229,-0.3171,-0.2996,-0.2596,-0.2277,-0.1657,-0.0977,-0.0397,0.0002,-0.0397,-0.1517,-0.2397,-0.2756,-0.2996]  InternalRulePriority=Speed  RndMeth=Simplest  InputSameDT=on
  Mux : Mux  Inputs=7
  Cn : Outport
  wires:
  alpha/1 -> Cn_del/1, Cn_der/1, Cn_dr/1, Cn_r/1, Cn_p/1, Cn_b/1, Cn_da/1
  Cn_b/1 -> Mux/1
  Cn_p/1 -> Mux/2
  Cn_r/1 -> Mux/3
  Cn_da/1 -> Mux/4
  Cn_del/1 -> Mux/5
  Cn_der/1 -> Mux/6
  Cn_dr/1 -> Mux/7
  Mux/1 -> Cn/1

== system HARV_6DoF_turn_mdl/Stability Derivatives/Longitudinal/CD ==
  Input : Inport
  CD0 : Lookup_n-D  NumberOfTableDimensions=1  BreakpointsForDimension1=[-0.2444,-0.1746,-0.1048,-0.0349,0.0349,0.1048,0.1746,0.2444,0.3143,0.3841,0.4540,0.5238,0.5937,0.6635,0.7333,0.8032,0.8730,0.9429,1.0127,1.0825,1.1524,1.2222,1.2921,1.3619,1.4317,1.5016,1.5714]  Table=|  InternalRulePriority=Speed  RndMeth=Simplest  InputSameDT=on
      | [    0.2273,
      |     0.1707,
      |     0.0748,
      |     0.0321,
      |     0.0279,
      |     0.0613,
      |     0.1540,
      |     0.2613,
      |     0.3639,
      |     0.4866,
      |     0.6440,
      |     0.8638,
      |     1.0856,
      |     1.2790,
      |     1.4764,
      |     1.6191,
      |     1.7460,
      |     1.8445,
      |     1.9240,
      |     1.9838,
      |     2.0283,
      |     2.0671,
      |     2.1136,
      |     2.1551,
      |     2.1736,
      |     2.1628,
      |     2.1282]
  CD_del : Lookup_n-D  NumberOfTableDimensions=1  BreakpointsForDimension1=[-0.2444,-0.1746,-0.1048,-0.0349,0.0349,0.1048,0.1746,0.2444,0.3143,0.3841,0.4540,0.5238,0.5937,0.6635,0.7333,0.8032,0.8730,0.9429,1.0127,1.0825,1.1524,1.2222,1.2921,1.3619,1.4317,1.5016,1.5714]  Table=|  InternalRulePriority=Speed  RndMeth=Simplest  InputSameDT=on
      | [   -0.1511,
      |    -0.1388,
      |    -0.1151,
      |    -0.0926,
      |    -0.0637,
      |    -0.0247,
      |     0.0249,
      |     0.0639,
      |     0.1129,
      |     0.1619,
      |     0.2061,
      |     0.2462,
      |     0.2828,
      |     0.3184,
      |     0.3372,
      |     0.3335,
      |     0.3147,
      |     0.2993,
      |     0.2950,
      |     0.2967,
      |     0.2979,
      |     0.2903,
      |     0.2092,
      |     0.1434,
      |     0.0971,
      |     0.0716,
      |     0.0648]
  CD_der : Lookup_n-D  NumberOfTableDimensions=1  BreakpointsForDimension1=[-0.2444,-0.1746,-0.1048,-0.0349,0.0349,0.1048,0.1746,0.2444,0.3143,0.3841,0.4540,0.5238,0.5937,0.6635,0.7333,0.8032,0.8730,0.9429,1.0127,1.0825,1.1524,1.2222,1.2921,1.3619,1.4317,1.5016,1.5714]  Table=|  InternalRulePriority=Speed  RndMeth=Simplest  InputSameDT=on
      | [   -0.1511,
      |    -0.1388,
      |    -0.1151,
      |    -0.0926,
      |    -0.0637,
      |    -0.0247,
      |     0.0249,
      |     0.0639,
      |     0.1129,
      |     0.1619,
      |     0.2061,
      |     0.2462,
      |     0.2828,
      |     0.3184,
      |     0.3372,
      |     0.3335,
      |     0.3147,
      |     0.2993,
      |     0.2950,
      |     0.2967,
      |     0.2979,
      |     0.2903,
      |     0.2092,
      |     0.1434,
      |     0.0971,
      |     0.0716,
      |     0.0648]
  CD_q : Lookup_n-D  NumberOfTableDimensions=1  BreakpointsForDimension1=[-0.2444,-0.1746,-0.1048,-0.0349,0.0349,0.1048,0.1746,0.2444,0.3143,0.3841,0.4540,0.5238,0.5937,0.6635,0.7333,0.8032,0.8730,0.9429,1.0127,1.0825,1.1524,1.2222,1.2921,1.3619,1.4317,1.5016,1.5714]  Table=|  InternalRulePriority=Speed  RndMeth=Simplest  InputSameDT=on
      | [    0.0000,
      |    -0.0000,
      |    -0.0050,
      |    -0.0446,
      |    -0.0476,
      |    -0.0038,
      |     0.0763,
      |     0.0096,
      |     0.0003,
      |    -0.0000,
      |    -0.0000,
      |    -0.0000,
      |    -0.0000,
      |     0.0000,
      |     0.0000,
      |     0.0000,
      |     0.0000,
      |    -0.0000,
      |     0.0000,
      |    -0.0000,
      |     0.0000,
      |    -0.0000,
      |    -0.0000,
      |    -0.0000,
      |    -0.0000,
      |     0.0000,
      |     0.0000
      | ]
  Mux : Mux
  Output : Outport
  wires:
  Input/1 -> CD_der/1, CD_del/1, CD_q/1, CD0/1
  CD_q/1 -> Mux/2
  CD_del/1 -> Mux/3
  CD_der/1 -> Mux/4
  Mux/1 -> Output/1
  CD0/1 -> Mux/1

== system HARV_6DoF_turn_mdl/Stability Derivatives/Longitudinal/CL ==
  alpha : Inport
  CL0 : Lookup_n-D  NumberOfTableDimensions=1  BreakpointsForDimension1=[-0.2444,-0.1746,-0.1048,-0.0349,0.0349,0.1048,0.1746,0.2444,0.3143,0.3841,0.4540,0.5238,0.5937,0.6635,0.7333,0.8032,0.8730,0.9429,1.0127,1.0825,1.1524,1.2222,1.2921,1.3619,1.4317,1.5016,1.5714]  Table=|  InternalRulePriority=Speed  RndMeth=Simplest  InputSameDT=on
      | [   -1.0386,
      |    -0.8809,
      |    -0.5513,
      |    -0.2162,
      |     0.1545,
      |     0.5609,
      |     0.9516,
      |     1.2417,
      |     1.3979,
      |     1.5310,
      |     1.6411,
      |     1.7772,
      |     1.8865,
      |     1.8894,
      |     1.8097,
      |     1.6856,
      |     1.5752,
      |     1.4601,
      |     1.3188,
      |     1.1712,
      |     1.0215,
      |     0.8589,
      |     0.6853,
      |     0.5295,
      |     0.3783,
      |     0.2293,
      |     0.0911]
  CL_del : Lookup_n-D  NumberOfTableDimensions=1  BreakpointsForDimension1=[-0.2444,-0.1746,-0.1048,-0.0349,0.0349,0.1048,0.1746,0.2444,0.3143,0.3841,0.4540,0.5238,0.5937,0.6635,0.7333,0.8032,0.8730,0.9429,1.0127,1.0825,1.1524,1.2222,1.2921,1.3619,1.4317,1.5016,1.5714]  Table=|  InternalRulePriority=Speed  RndMeth=Simplest  InputSameDT=on
      | [    0.2885,
      |     0.3040,
      |     0.3323,
      |     0.3580,
      |     0.3872,
      |     0.4117,
      |     0.4101,
      |     0.3940,
      |     0.3797,
      |     0.3602,
      |     0.3422,
      |     0.3384,
      |     0.3358,
      |     0.3184,
      |     0.2726,
      |     0.2039,
      |     0.1298,
      |     0.0893,
      |     0.0598,
      |     0.0337,
      |     0.0068,
      |    -0.0211,
      |    -0.0632,
      |    -0.1027,
      |    -0.1302,
      |    -0.1424,
      |    -0.1419]
  CL_der : Lookup_n-D  NumberOfTableDimensions=1  BreakpointsForDimension1=[-0.2444,-0.1746,-0.1048,-0.0349,0.0349,0.1048,0.1746,0.2444,0.3143,0.3841,0.4540,0.5238,0.5937,0.6635,0.7333,0.8032,0.8730,0.9429,1.0127,1.0825,1.1524,1.2222,1.2921,1.3619,1.4317,1.5016,1.5714]  Table=|  InternalRulePriority=Speed  RndMeth=Simplest  InputSameDT=on
      | [    0.2885,
      |     0.3040,
      |     0.3323,
      |     0.3580,
      |     0.3872,
      |     0.4117,
      |     0.4101,
      |     0.3940,
      |     0.3797,
      |     0.3602,
      |     0.3422,
      |     0.3384,
      |     0.3358,
      |     0.3184,
      |     0.2726,
      |     0.2039,
      |     0.1298,
      |     0.0893,
      |     0.0598,
      |     0.0337,
      |     0.0068,
      |    -0.0211,
      |    -0.0632,
      |    -0.1027,
      |    -0.1302,
      |    -0.1424,
      |    -0.1419]
  CL_q : Lookup_n-D  NumberOfTableDimensions=1  BreakpointsForDimension1=[-0.2444,-0.1746,-0.1048,-0.0349,0.0349,0.1048,0.1746,0.2444,0.3143,0.3841,0.4540,0.5238,0.5937,0.6635,0.7333,0.8032,0.8730,0.9429,1.0127,1.0825,1.1524,1.2222,1.2921,1.3619,1.4317,1.5016,1.5714]  Table=|  InternalRulePriority=Speed  RndMeth=Simplest  InputSameDT=on
      | [
      |     4.5082,
      |     4.5082,
      |     4.5082,
      |     4.5157,
      |     4.3807,
      |     3.9609,
      |     3.6285,
      |     3.4311,
      |     3.3736,
      |     3.4686,
      |     3.6011,
      |     3.9609,
      |     5.0929,
      |     6.8722,
      |     8.4666,
      |     9.1463,
      |     7.5469,
      |     5.9476,
      |     5.2779,
      |     5.0380,
      |     4.9480,
      |     4.9480,
      |     4.8680,
      |     4.7281,
      |     4.5682,
      |     4.3882,
      |     4.1483]
  Mux : Mux
  CL_derivatives : Outport
  wires:
  alpha/1 -> CL_del/1, CL_der/1, CL_q/1, CL0/1
  CL_q/1 -> Mux/2
  CL_del/1 -> Mux/3
  CL_der/1 -> Mux/4
  Mux/1 -> CL_derivatives/1
  CL0/1 -> Mux/1

== system HARV_6DoF_turn_mdl/Stability Derivatives/Longitudinal/CM ==
  Input : Inport
  CM0 : Lookup_n-D  NumberOfTableDimensions=1  BreakpointsForDimension1=[-0.2444,-0.1746,-0.1048,-0.0349,0.0349,0.1048,0.1746,0.2444,0.3143,0.3841,0.4540,0.5238,0.5937,0.6635,0.7333,0.8032,0.8730,0.9429,1.0127,1.0825,1.1524,1.2222,1.2921,1.3619,1.4317,1.5016,1.5714]  Table=|  InternalRulePriority=Speed  RndMeth=Simplest  InputSameDT=on
      | [    0.0963,
      |     0.0807,
      |     0.0554,
      |     0.0281,
      |     0.0051,
      |    -0.0066,
      |    -0.0164,
      |    -0.0160,
      |    -0.0586,
      |    -0.0842,
      |    -0.0853,
      |    -0.1056,
      |    -0.1171,
      |    -0.1101,
      |    -0.1141,
      |    -0.1184,
      |    -0.1018,
      |    -0.1461,
      |    -0.2283,
      |    -0.3516,
      |    -0.4263,
      |    -0.4769,
      |    -0.6017,
      |    -0.5635,
      |    -0.5477,
      |    -0.5700,
      |    -0.5880]
  CM_del : Lookup_n-D  NumberOfTableDimensions=1  BreakpointsForDimension1=[-0.2444,-0.1746,-0.1048,-0.0349,0.0349,0.1048,0.1746,0.2444,0.3143,0.3841,0.4540,0.5238,0.5937,0.6635,0.7333,0.8032,0.8730,0.9429,1.0127,1.0825,1.1524,1.2222,1.2921,1.3619,1.4317,1.5016,1.5714]  Table=|  InternalRulePriority=Speed  RndMeth=Simplest  InputSameDT=on
      | [   -0.3704,
      |    -0.3774,
      |    -0.3912,
      |    -0.4064,
      |    -0.4271,
      |    -0.4484,
      |    -0.4587,
      |    -0.4607,
      |    -0.4611,
      |    -0.4584,
      |    -0.4581,
      |    -0.4575,
      |    -0.4466,
      |    -0.4212,
      |    -0.3660,
      |    -0.2896,
      |    -0.2148,
      |    -0.1934,
      |    -0.1736,
      |    -0.1331,
      |    -0.0788,
      |    -0.0466,
      |    -0.0447,
      |    -0.1015,
      |    -0.1347,
      |    -0.1349,
      |    -0.1661]
  CM_der : Lookup_n-D  NumberOfTableDimensions=1  BreakpointsForDimension1=[-0.2444,-0.1746,-0.1048,-0.0349,0.0349,0.1048,0.1746,0.2444,0.3143,0.3841,0.4540,0.5238,0.5937,0.6635,0.7333,0.8032,0.8730,0.9429,1.0127,1.0825,1.1524,1.2222,1.2921,1.3619,1.4317,1.5016,1.5714]  Table=|  InternalRulePriority=Speed  RndMeth=Simplest  InputSameDT=on
      | [
      |    -0.3704,
      |    -0.3774,
      |    -0.3912,
      |    -0.4064,
      |    -0.4271,
      |    -0.4484,
      |    -0.4587,
      |    -0.4607,
      |    -0.4611,
      |    -0.4584,
      |    -0.4581,
      |    -0.4575,
      |    -0.4466,
      |    -0.4212,
      |    -0.3660,
      |    -0.2896,
      |    -0.2148,
      |    -0.1934,
      |    -0.1736,
      |    -0.1331,
      |    -0.0788,
      |    -0.0466,
      |    -0.0447,
      |    -0.1015,
      |    -0.1347,
      |    -0.1349,
      |    -0.1661]
  CM_q : Lookup_n-D  NumberOfTableDimensions=1  BreakpointsForDimension1=[-0.2444,-0.1746,-0.1048,-0.0349,0.0349,0.1048,0.1746,0.2444,0.3143,0.3841,0.4540,0.5238,0.5937,0.6635,0.7333,0.8032,0.8730,0.9429,1.0127,1.0825,1.1524,1.2222,1.2921,1.3619,1.4317,1.5016,1.5714]  Table=|  InternalRulePriority=Speed  RndMeth=Simplest  InputSameDT=on
      | [   -4.9730,
      |    -4.9730,
      |    -4.9730,
      |    -4.9580,
      |    -4.8905,
      |    -4.6306,
      |    -4.3383,
      |    -4.1458,
      |    -4.3333,
      |    -4.7481,
      |    -5.0505,
      |    -5.8627,
      |    -8.4566,
      |   -11.7728,
      |    -7.6019,
      |     1.0346,
      |     2.4740,
      |     1.0346,
      |    -1.1245,
      |    -3.7235,
      |    -5.7827,
      |    -5.6227,
      |    -5.4628,
      |    -5.3029,
      |    -5.1029,
      |    -4.8830,
      |    -4.7231]
  Mux : Mux
  Output : Outport
  wires:
  Input/1 -> CM_q/1, CM0/1, CM_der/1, CM_del/1
  CM_q/1 -> Mux/2
  CM_del/1 -> Mux/3
  CM_der/1 -> Mux/4
  Mux/1 -> Output/1
  CM0/1 -> Mux/1
